simulink model "lifter"  (R2018b)
settings: Solver=VariableStepAuto  StartTime=0.0  StopTime=10.0  RelTol=1e-3
libraries: simulink x1
settings Model: Creator=Hiro  LastModifiedBy=Hiro

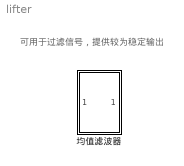
== system lifter ==
  note: 可用于过滤信号，提供较为稳定输出
  均值滤波器 : Subsystem

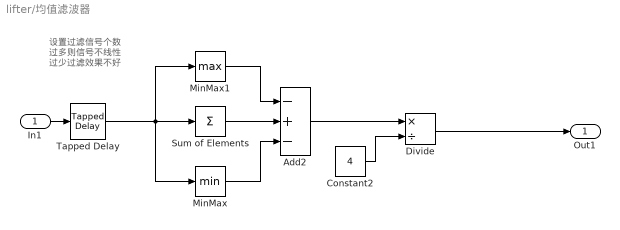
== system lifter/均值滤波器 ==
  note: 设置过滤信号个数
      |
      | 过多则信号不线性
      | 过少过滤效果不好
  In1 : Inport
  Add2 : Sum  Inputs=-+-
  Constant2 : Constant  Value=4  OutDataTypeStr=uint8  SampleTime=-1
  Divide : Product  Inputs=*/
  MinMax : MinMax
  MinMax1 : MinMax  Function=max
  Sum of Elements : Sum  Inputs=+
  Tapped Delay : simulink/Discrete/Tapped Delay  vinit=0.0  samptime=-1  NumDelays=4  DelayOrder=Oldest  includeCurrent=off
  Out1 : Outport
  wires:
  Tapped Delay/1 -> Sum of Elements/1, MinMax1/1, MinMax/1
  Sum of Elements/1 -> Add2/2
  Constant2/1 -> Divide/2
  Divide/1 -> Out1/1
  MinMax1/1 -> Add2/1
  MinMax/1 -> Add2/3
  Add2/1 -> Divide/1
  In1/1 -> Tapped Delay/1
